simulink library "forceTether"  (R2018b)
settings: Solver=VariableStepAuto  StartTime=0.0  StopTime=10.0  RelTol=1e-3
values from neighbouring files (symbols this model uses):
  b = zeta*(2*sqrt(k*ms))    [Platform.m]    (also in sprungODE.m = system_param.b)
  k = E*A/lus    (= 34906585039.9)    [Platform.m]    (also in sprungODE.m = system_param.k)
undefined symbols (not defined in the file or in its folder): anchorPosition, cmDistance, unstretched
settings Model: Creator=embeato2  LastModifiedBy=embeato2

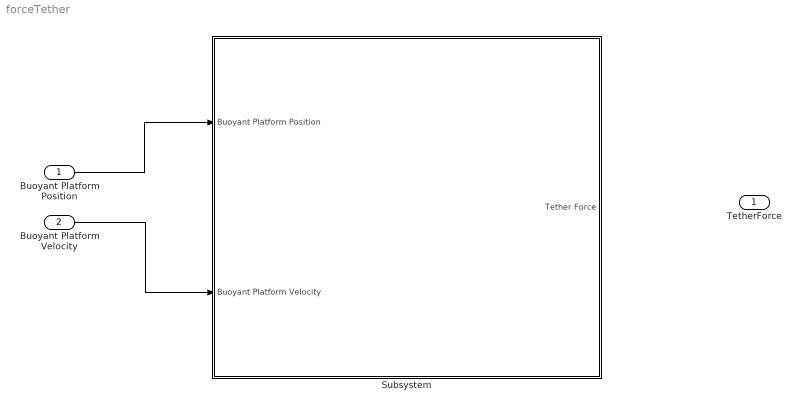
== system forceTether ==
  Buoyant Platform Position : Inport
  Buoyant Platform Velocity : Inport  Port=2
  Subsystem : Subsystem
  TetherForce : Outport
  wires:
  Buoyant Platform Position/1 -> Subsystem/1(Buoyant Platform Position)
  Buoyant Platform Velocity/1 -> Subsystem/2(Buoyant Platform Velocity)
  ? -> TetherForce/1

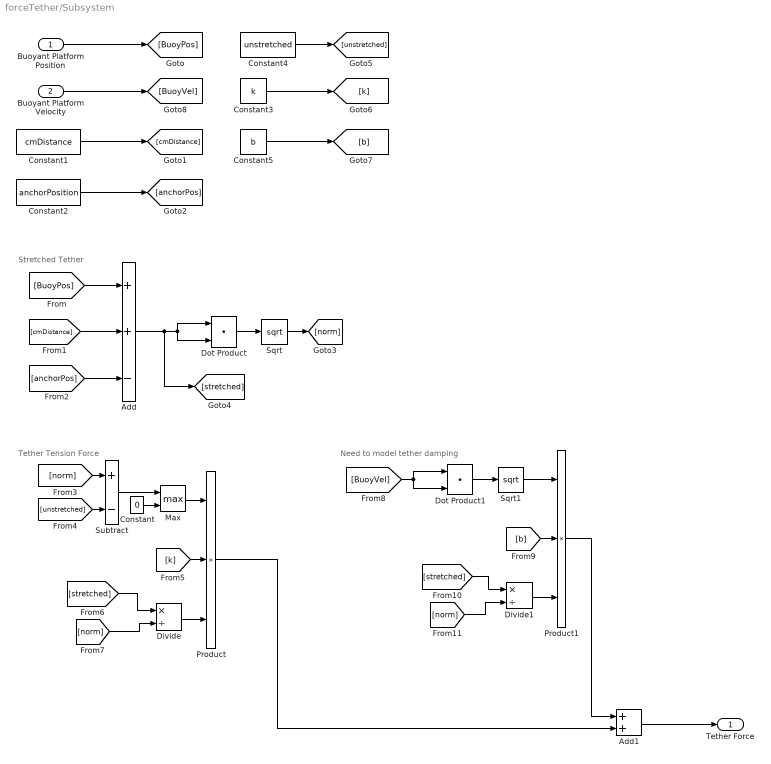
== system forceTether/Subsystem ==
  note: Stretched Tether
  note: Tether Tension Force
  note: Need to model tether damping
  Buoyant Platform Position : Inport
  Buoyant Platform Velocity : Inport  Port=2
  Add : Sum  Inputs=++-
  Add1 : Sum
  Constant : Constant  Value=0
  Constant1 : Constant  Value=cmDistance
  Constant2 : Constant  Value=anchorPosition
  Constant3 : Constant  Value=k
  Constant4 : Constant  Value=unstretched
  Constant5 : Constant  Value=b
  Divide : Product  Inputs=*/
  Divide1 : Product  Inputs=*/
  Dot Product : DotProduct  InputSameDT=on  OutDataTypeStr=Inherit: Inherit via internal rule
  Dot Product1 : DotProduct  InputSameDT=on  OutDataTypeStr=Inherit: Inherit via internal rule
  Max : MinMax  Function=max  Inputs=2
  Product : Product  Inputs=3
  Product1 : Product  Inputs=3
  Sqrt : Sqrt  SaturateOnIntegerOverflow=on
  Sqrt1 : Sqrt  SaturateOnIntegerOverflow=on
  Subtract : Sum  Inputs=+-
  Tether Force : Outport
  wires:
  Constant2/1 -> [anchorPos]
  [anchorPos] -> Add/3
  [stretched] -> Divide/1
  [unstretched] -> Subtract/2
  Divide/1 -> Product/3
  [k] -> Product/2
  [norm] -> Divide/2
  Add/1 -> [stretched], Dot Product/1, Dot Product/2
  Subtract/1 -> Max/1
  Constant1/1 -> [cmDistance]
  Buoyant Platform Position/1 -> [BuoyPos]
  Buoyant Platform Velocity/1 -> [BuoyVel]
  [norm] -> Subtract/1
  [cmDistance] -> Add/2
  [BuoyPos] -> Add/1
  Sqrt/1 -> [norm]
  Constant/1 -> Max/2
  Max/1 -> Product/1
  Dot Product/1 -> Sqrt/1
  Constant5/1 -> [b]
  Constant3/1 -> [k]
  Constant4/1 -> [unstretched]
  Dot Product1/1 -> Sqrt1/1
  [BuoyVel] -> Dot Product1/1, Dot Product1/2
  Sqrt1/1 -> Product1/1
  [norm] -> Divide1/2
  [b] -> Product1/2
  Divide1/1 -> Product1/3
  [stretched] -> Divide1/1
  Add1/1 -> Tether Force/1
  Product1/1 -> Add1/1
  Product/1 -> Add1/2
